simulink model "PID_controller"  (R2021a)
settings: configuration reference "Controller_Config_sim" (kept outside this file)
undefined symbols (not defined in the file or in its folder): dphi_gain, dtheta_gain, phi_gain, theta_gain, Volt_Limit
libraries: angle_lib x6
settings Model: DataDictionary=sys_PID_data.sldd  Creator=tshintai  LastModifiedBy=tshintai
settings ConfigSetRef: SourceName=Controller_Config_sim

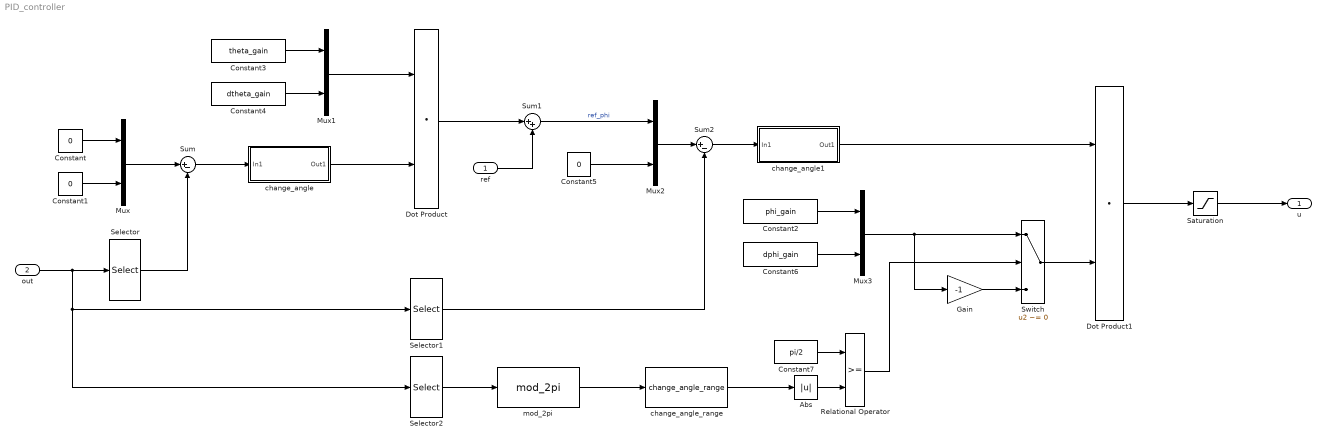
== system PID_controller ==
  ref : Inport
  out : Inport  Port=2  PortDimensions=4
  Abs : Abs
  Constant : Constant  Value=0
  Constant1 : Constant  Value=0
  Constant2 : Constant  Value=phi_gain
  Constant3 : Constant  Value=theta_gain
  Constant4 : Constant  Value=dtheta_gain
  Constant5 : Constant  Value=0
  Constant6 : Constant  Value=dphi_gain
  Constant7 : Constant  Value=pi/2
  Dot Product : DotProduct  InputSameDT=on  OutDataTypeStr=Inherit: Inherit via internal rule
  Dot Product1 : DotProduct  InputSameDT=on  OutDataTypeStr=Inherit: Inherit via internal rule
  Gain : Gain  Gain=-1
  Mux{,1..3} (4 alike) : Mux  Inputs=2
  Relational Operator : RelationalOperator  OutDataTypeStr=boolean  RndMeth=Simplest
  Saturation : Saturate  UpperLimit=Volt_Limit  LowerLimit=-Volt_Limit
  Selector : Selector  InputPortWidth=4  IndexOptions=Index vector (dialog)  Indices=[1 3]  OutputSizes=1
  Selector1 : Selector  InputPortWidth=4  IndexOptions=Index vector (dialog)  Indices=[2 4]  OutputSizes=1
  Selector2 : Selector  InputPortWidth=4  IndexOptions=Index vector (dialog)  Indices=[2]  OutputSizes=1
  Sum : Sum  Inputs=|+-
  Sum1 : Sum  Inputs=|++
  Sum2 : Sum  Inputs=|+-
  Switch : Switch  Criteria=u2 ~= 0
  change_angle : Subsystem
  change_angle1 : Subsystem
  change_angle_range : angle_lib/change_angle_range  SystemSampleTime=-1  VariantActivationTime=update diagram  Latency=0  AutoFrameSizeCalculation=off
  mod_2pi : angle_lib/mod_2pi  SystemSampleTime=-1  VariantActivationTime=update diagram  Latency=0  AutoFrameSizeCalculation=off
  u : Outport
  wires:
  Constant/1 -> Mux/1
  Sum/1 -> change_angle/1(In1)
  change_angle/1(Out1) -> Dot Product/2
  Constant1/1 -> Mux/2
  out/1 -> Selector2/1, Selector1/1, Selector/1
  Mux/1 -> Sum/1
  Selector/1 -> Sum/2
  Mux1/1 -> Dot Product/1
  Constant4/1 -> Mux1/2
  Constant3/1 -> Mux1/1
  Dot Product/1 -> Sum1/1
  Constant5/1 -> Mux2/2
  ref/1 -> Sum1/2
  Sum1/1 -> Mux2/1  "ref_phi"
  Selector1/1 -> Sum2/2
  Sum2/1 -> change_angle1/1(In1)
  Mux2/1 -> Sum2/1
  change_angle1/1(Out1) -> Dot Product1/1
  Dot Product1/1 -> Saturation/1
  Saturation/1 -> u/1
  Constant2/1 -> Mux3/1
  Mux3/1 -> Switch/1, Gain/1
  Constant6/1 -> Mux3/2
  Selector2/1 -> mod_2pi/1
  Constant7/1 -> Relational Operator/1
  Abs/1 -> Relational Operator/2
  Relational Operator/1 -> Switch/2
  Gain/1 -> Switch/3
  Switch/1 -> Dot Product1/2
  mod_2pi/1 -> change_angle_range/1
  change_angle_range/1 -> Abs/1

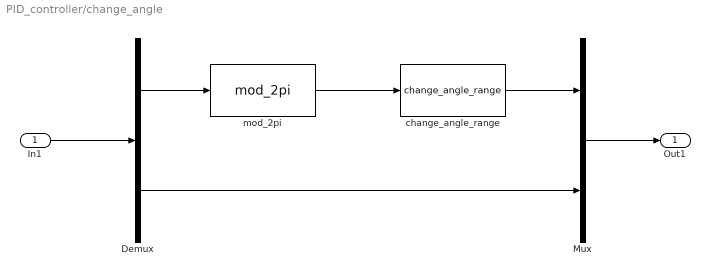
== system PID_controller/change_angle ==
  In1 : Inport
  Demux : Demux  Outputs=2
  Mux : Mux  Inputs=2
  change_angle_range : angle_lib/change_angle_range  SystemSampleTime=-1  VariantActivationTime=update diagram  Latency=0  AutoFrameSizeCalculation=off
  mod_2pi : angle_lib/mod_2pi  SystemSampleTime=-1  VariantActivationTime=update diagram  Latency=0  AutoFrameSizeCalculation=off
  Out1 : Outport
  wires:
  In1/1 -> Demux/1
  Demux/1 -> mod_2pi/1
  mod_2pi/1 -> change_angle_range/1
  change_angle_range/1 -> Mux/1
  Demux/2 -> Mux/2
  Mux/1 -> Out1/1

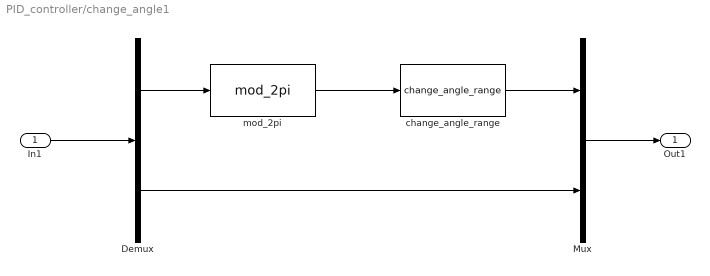
== system PID_controller/change_angle1 ==
  In1 : Inport
  Demux : Demux  Outputs=2
  Mux : Mux  Inputs=2
  change_angle_range : angle_lib/change_angle_range  SystemSampleTime=-1  VariantActivationTime=update diagram  Latency=0  AutoFrameSizeCalculation=off
  mod_2pi : angle_lib/mod_2pi  SystemSampleTime=-1  VariantActivationTime=update diagram  Latency=0  AutoFrameSizeCalculation=off
  Out1 : Outport
  wires:
  Mux/1 -> Out1/1
  Demux/2 -> Mux/2
  change_angle_range/1 -> Mux/1
  mod_2pi/1 -> change_angle_range/1
  Demux/1 -> mod_2pi/1
  In1/1 -> Demux/1
